simulink subsystem "cvrs_diastole_coefficients"  (R2020b)
settings: Solver=VariableStepAuto  StartTime=0.0  StopTime=10.0  RelTol=1e-3
settings Model: Creator=RH  LastModifiedBy=Marco

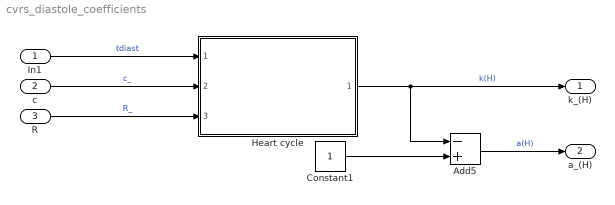
== system cvrs_diastole_coefficients ==
  In1 : Inport  Unit=second
  c : Inport  Port=2  Unit=liter/mmHg
  R : Inport  Port=3  Unit=mmHg*minute/liter
  Add5 : Sum  Inputs=-+
  Constant1 : Constant
  Heart cycle : Subsystem  ReferencedSubsystem=heart_cycle
  k_(H) : Outport
  a_(H) : Outport  Port=2
  wires:
  Heart cycle/1 -> Add5/1, k_(H)/1  "k(H)"
  Constant1/1 -> Add5/2
  Add5/1 -> a_(H)/1  "a(H)"
  R/1 -> Heart cycle/3  "R_"
  In1/1 -> Heart cycle/1  "tdiast"
  c/1 -> Heart cycle/2  "c_"
